simulink model "MCU_vectorControl_dsPIC33CK_LVMC_FW_teknicMotor"  (R2018a)
settings: Solver=FixedStepDiscrete  StartTime=0.0  StopTime=10.0  FixedStep=50e-6  RelTol=1e-3  EnableMultiTasking=on
undefined symbols (not defined in the file): A0, A4, AN0, AN1, B0, B2, Bias1, Bias2, C12, C13, C14, C7, control, D11, D12, D13, D14, D5, D6, D7, DiscIntNeverNeededParam, inverter, Max, MaxPer, model, ms, NumBits1, NumBits2, P20, P32, P55, P60, P61, P62, P69, P70, P71, P75, P76, P77, P78, Pin, pmsm, PosRange1, PosRange2, PWM1max, Resol, s, Slope1, Slope2, us
libraries: simulink x43, MCHP_Blockset x23
(part 4 of 4)

== system MCU_vectorControl_dsPIC33CK_LVMC_FW_teknicMotor/BOARD dsPIC33CK LVMC/Timing Analysis/Downsample Averaged2 ==
  note: DownSample & Average by changing data scaling
  In1 : Inport
  Compare To Constant : simulink/Logic and Bit Operations/Compare To Constant  relop===  const=1  OutDataTypeStr=boolean
  Counter Limited : simulink/Sources/Counter Limited  uplimit=DownSample-1  tsamp=-1
  Data Type Duplicate : DataTypeDuplicate
  Data Type Propagation : simulink/Signal Attributes/Data Type Propagation  PropDataType=fixdt(1, 16)  IfRefDouble=double  IfRefSingle=single  IsSigned=IsSigned1 or IsSigned2  NumBitsBase=NumBits1+NumBits2  NumBitsMult=1  NumBitsAdd=0  NumBitsAllowFinal=1:128  PropScaling=2^-10  ValuesUsedBestPrec=[5 -7]  SlopeBase=Slope1  SlopeMult=1  SlopeAdd=0  BiasBase=Bias1  BiasMult=1  BiasAdd=0
      settings: SourceProductName=Simulink  SourceProductBaseCode=SL
  Data Type Propagation1 : simulink/Signal Attributes/Data Type Propagation  PropDataType=fixdt(1, 16)  IfRefDouble=double  IfRefSingle=single  IsSigned=IsSigned1 or IsSigned2  NumBitsBase=NumBits1+NumBits2  NumBitsMult=1  NumBitsAdd=0  NumBitsAllowFinal=1:128  PropScaling=2^-10  ValuesUsedBestPrec=[5 -7]  SlopeBase=PosRange1  SlopeMult=1  SlopeAdd=0  BiasBase=Bias1  BiasMult=1  BiasAdd=0
      settings: SourceProductName=Simulink  SourceProductBaseCode=SL
  Discrete-Time Integrator : DiscreteIntegrator  IntegratorMethod=Accumulation: Backward Euler  gainval=1  ExternalReset=sampled level  SampleTime=-1  OutDataTypeStr=Inherit: Inherit via back propagation  ICPrevOutput=DiscIntNeverNeededParam  ICPrevScaledInput=DiscIntNeverNeededParam
  Gain : Gain  Gain=1/DownSample  OutDataTypeStr=Inherit: Inherit via back propagation
  Gain1 : Gain  Gain=1/DownSample  OutDataTypeStr=Inherit: Inherit via back propagation
  Rate Transition1 : RateTransition  Deterministic=off  OutPortSampleTime=[InputSampleTime * DownSample]
  Rate Transition3 : RateTransition  OutPortSampleTime=[InputSampleTime * DownSample]
  Terminator : Terminator
  Out1 : Outport
  wires:
  Rate Transition3/1 -> Gain1/1, Gain/1
  In1/1 -> Discrete-Time Integrator/1, Rate Transition1/1, Data Type Propagation/2, Data Type Propagation/1
  Compare To Constant/1 -> Discrete-Time Integrator/2
  Discrete-Time Integrator/1 -> Data Type Propagation/3, Rate Transition3/1
  Counter Limited/1 -> Compare To Constant/1
  Gain/1 -> Data Type Duplicate/2, Out1/1
  Rate Transition1/1 -> Data Type Propagation1/2, Data Type Propagation1/1, Data Type Duplicate/1
  Gain1/1 -> Data Type Propagation1/3, Terminator/1

== system MCU_vectorControl_dsPIC33CK_LVMC_FW_teknicMotor/Control law/Speed control/Current Control ==
  idqref : Inport
  idq : Inport  Port=2
  Data Type Duplicate : DataTypeDuplicate  NumInputPorts=3
  Data Type Propagation : simulink/Signal Attributes/Data Type Propagation  PropDataType=fixdt(1, 16)  IfRefDouble=double  IfRefSingle=single  IsSigned=IsSigned1 or IsSigned2  NumBitsBase=max([NumBits1 NumBits2])  NumBitsMult=1  NumBitsAdd=0  NumBitsAllowFinal=1:128  PropScaling=2^-(15-ceil(log2(2*inverter.iMax)))  ValuesUsedBestPrec=[5 -7]  SlopeBase=max([PosRange1 PosRange2])  SlopeMult=2  SlopeAdd=0  BiasBase=Bias1  BiasMult=1  BiasAdd=0
      settings: SourceProductName=Simulink  SourceProductBaseCode=SL
  Gain : Gain  Gain=control.kE(2)  OutDataTypeStr=Inherit: Inherit via back propagation  SaturateOnIntegerOverflow=on
  Gain1 : Gain  Gain=control.kE(1)  OutDataTypeStr=Inherit: Inherit via back propagation  SaturateOnIntegerOverflow=on
  Integrator : Subsystem
  Sum : Sum  Inputs=|--  OutDataTypeStr=Inherit: Inherit via back propagation  SaturateOnIntegerOverflow=on
  Sum3 : Sum  Inputs=|+-  OutDataTypeStr=Inherit: Inherit via back propagation  SaturateOnIntegerOverflow=on
  v : Outport
  wires:
  Sum/1 -> v/1, Data Type Duplicate/1
  Integrator/1(Out1) -> Gain/1
  idqref/1 -> Sum3/1, Data Type Propagation/1
  Sum3/1 -> Integrator/1(In1), Data Type Propagation/3
  idq/1 -> Sum3/2, Gain1/1, Data Type Propagation/2
  Gain/1 -> Sum/1, Data Type Duplicate/2
  Gain1/1 -> Sum/2, Data Type Duplicate/3

== system MCU_vectorControl_dsPIC33CK_LVMC_FW_teknicMotor/Control law/Speed control/Mechanical Control ==
  omref : Inport
  om : Inport  Port=2
  isat : Inport  Port=3
  Clamping circuit : Subsystem
  Constant : Constant  Value=0  OutMax=model.iMax  OutDataTypeStr=fixdt(1,16)
  Data Type Duplicate1 : DataTypeDuplicate
  Data Type Propagation : simulink/Signal Attributes/Data Type Propagation  PropDataType=fixdt(1, 16)  IfRefDouble=double  IfRefSingle=single  IsSigned=IsSigned1 or IsSigned2  NumBitsBase=max([NumBits1 NumBits2])  NumBitsMult=1  NumBitsAdd=0  NumBitsAllowFinal=1:128  PropScaling=2^-(15-ceil(log2(2*pmsm.omMax)))  ValuesUsedBestPrec=[5 -7]  SlopeBase=max([PosRange1 PosRange2])  SlopeMult=2  SlopeAdd=0  BiasBase=Bias1  BiasMult=1  BiasAdd=0
      settings: SourceProductName=Simulink  SourceProductBaseCode=SL
  Delay : Delay  DelayLength=1
  Gain : Gain  Gain=control.kM(2)  OutDataTypeStr=Inherit: Inherit via back propagation  SaturateOnIntegerOverflow=on
  Gain1 : Gain  Gain=control.kM(1)  OutMax=model.iMax  OutDataTypeStr=fixdt(1,16)  SaturateOnIntegerOverflow=on
  Integrator : Subsystem
  Saturation Dynamic : simulink/Discontinuities/Saturation Dynamic  OutMin=[]  OutMax=[]  OutDataTypeStr=Inherit: Same as second input  OutDataType=fixdt(1, 16)  OutScaling=2^-10  DoSatur=off
  Sum : Sum  Inputs=|--  OutMax=2*model.iMax  OutDataTypeStr=fixdt(1,16)  SaturateOnIntegerOverflow=on
  Sum1 : Sum  Inputs=|+-  OutDataTypeStr=Inherit: Inherit via back propagation
  Sum2 : Sum  Inputs=|-+  SaturateOnIntegerOverflow=on  OutDataTypeStr=Inherit: Same as first input
  iqref : Outport
  wires:
  Saturation Dynamic/1 -> Sum2/1, iqref/1
  Sum/1 -> Sum2/2, Saturation Dynamic/2
  Gain/1 -> Sum/1
  om/1 -> Sum1/2, Gain1/1, Data Type Propagation/2, Data Type Duplicate1/2
  Sum1/1 -> Integrator/1(In1), Clamping circuit/2(preIntegrator), Data Type Propagation/3
  omref/1 -> Sum1/1, Data Type Propagation/1, Data Type Duplicate1/1
  Clamping circuit/1(Clamp) -> Integrator/Enable
  Sum2/1 -> Clamping circuit/1(Saturation)
  Integrator/1(Out1) -> Gain/1
  Gain1/1 -> Sum/2
  isat/1 -> Delay/1
  Delay/1 -> Saturation Dynamic/1
  Constant/1 -> Saturation Dynamic/3

== system MCU_vectorControl_dsPIC33CK_LVMC_FW_teknicMotor/Control law/Speed control/Subsystem2 ==
  om : Inport
  iref : Inport  Port=2
  Imax : Inport  Port=3
  Subsystem6 : Subsystem
  decision1 : Subsystem
  idq : Outport  VectorParamsAs1DForOutWhenUnconnected=on
  isat : Outport  Port=2  VectorParamsAs1DForOutWhenUnconnected=on
  wires:
  om/1 -> Subsystem6/2(om)
  Imax/1 -> Subsystem6/1(Imax), decision1/1(Imax)
  iref/1 -> decision1/2(iqref)
  decision1/1(idq) -> idq/1
  Subsystem6/2(i2(w)) -> decision1/4(i2(w))
  Subsystem6/3(i4(w)) -> decision1/5(i3(w))
  Subsystem6/1(i1(w)) -> decision1/3(i1(w))
  Subsystem6/4(a(w)) -> decision1/6(a(w))
  Subsystem6/5(b(w)) -> decision1/7(b(w))
  Subsystem6/6(c(w)) -> decision1/8(c(w))
  decision1/2(isat) -> isat/1
  Subsystem6/7(delta) -> decision1/9(delta)

== system MCU_vectorControl_dsPIC33CK_LVMC_FW_teknicMotor/Control law/Voltage Saturation/Norm L3 ==
  In1 : Inport
  Data Type Propagation : simulink/Signal Attributes/Data Type Propagation  PropDataType=fixdt(1, 16)  IfRefDouble=double  IfRefSingle=single  IsSigned=IsSigned1 or IsSigned2  NumBitsBase=max([NumBits1 NumBits2])  NumBitsMult=1  NumBitsAdd=0  NumBitsAllowFinal=1:128  PropScaling=2^-10  ValuesUsedBestPrec=[5 -7]  SlopeBase=Slope1/Slope2  SlopeMult=1  SlopeAdd=0  BiasBase=max([Bias1 Bias2])  BiasMult=1  BiasAdd=0
      settings: SourceProductName=Simulink  SourceProductBaseCode=SL
  Data Type Propagation1 : simulink/Signal Attributes/Data Type Propagation  PropDataType=fixdt(1, 16)  IfRefDouble=double  IfRefSingle=single  IsSigned=IsSigned1 or IsSigned2  NumBitsBase=max([NumBits1 NumBits2])  NumBitsMult=1  NumBitsAdd=0  NumBitsAllowFinal=1:128  PropScalingMode=Specify via dialog  PropScaling=2^-(15-ceil(log2(2*model.vMax)))  ValuesUsedBestPrec=[5 -7]  SlopeBase=Slope1/Slope2  SlopeMult=1  SlopeAdd=0  BiasBase=max([Bias1 Bias2])  BiasMult=1  BiasAdd=0
      settings: SourceProductName=Simulink  SourceProductBaseCode=SL
  Dot Product : DotProduct  OutDataTypeStr=Inherit: Inherit via back propagation  SaturateOnIntegerOverflow=on  InputSameDT=on
  Sqrt : Sqrt  OutputSignalType=real  OutDataTypeStr=Inherit: Inherit via back propagation  SaturateOnIntegerOverflow=on
  y : Outport  VectorParamsAs1DForOutWhenUnconnected=on
  wires:
  Dot Product/1 -> Data Type Propagation/3, Sqrt/1
  Sqrt/1 -> y/1, Data Type Propagation1/3
  In1/1 -> Dot Product/1, Dot Product/2, Data Type Propagation/2, Data Type Propagation/1, Data Type Propagation1/1, Data Type Propagation1/2

== system MCU_vectorControl_dsPIC33CK_LVMC_FW_teknicMotor/Control law/Speed control/Current Control/Integrator ==
  In1 : Inport
  Data Type Propagation : simulink/Signal Attributes/Data Type Propagation  PropDataType=fixdt(1, 16)  IfRefDouble=single  IfRefSingle=single  IsSigned=IsSigned1 or IsSigned2  NumBitsBase=NumBits1+NumBits2  NumBitsMult=1  NumBitsAdd=0  NumBitsAllowFinal=1:128  PropScalingMode=Specify via dialog  PropScaling=2^-23  ValuesUsedBestPrec=[5 -7]  SlopeBase=min([Slope1 Slope2])  SlopeMult=1  SlopeAdd=0  BiasBase=Bias1  BiasMult=1  BiasAdd=0
      settings: SourceProductName=Simulink  SourceProductBaseCode=SL
  Discrete-Time Integrator : DiscreteIntegrator  SampleTime=-1  OutDataTypeStr=Inherit: Inherit via back propagation  SaturateOnIntegerOverflow=on  ICPrevOutput=DiscIntNeverNeededParam  ICPrevScaledInput=DiscIntNeverNeededParam
  Out1 : Outport
  wires:
  Discrete-Time Integrator/1 -> Out1/1, Data Type Propagation/3
  In1/1 -> Data Type Propagation/1, Data Type Propagation/2, Discrete-Time Integrator/1

== system MCU_vectorControl_dsPIC33CK_LVMC_FW_teknicMotor/Control law/Speed control/Mechanical Control/Clamping circuit ==
  note: The clamping enable or disable the integral action.
  Saturation : Inport  DisableCoverage=on
  preIntegrator : Inport  DisableCoverage=on  Port=2
  Compare To Zero1 : simulink/Logic and Bit Operations/Compare To Zero  relop=<=  OutDataTypeStr=boolean
  Delay : Delay  DelayLength=1  InitialCondition=0
  Multiply : Product  SaturateOnIntegerOverflow=on  OutDataTypeStr=Inherit: Same as first input
  Clamp : Outport  DisableCoverage=on
  wires:
  Delay/1 -> Multiply/1
  Saturation/1 -> Delay/1
  Multiply/1 -> Compare To Zero1/1
  preIntegrator/1 -> Multiply/2
  Compare To Zero1/1 -> Clamp/1

== system MCU_vectorControl_dsPIC33CK_LVMC_FW_teknicMotor/Control law/Speed control/Mechanical Control/Integrator ==
  In1 : Inport
  Enable : EnablePort
  Discrete-Time Integrator : DiscreteIntegrator  SampleTime=-1  OutDataTypeStr=fixdt(1,32,20)  SaturateOnIntegerOverflow=on  ICPrevOutput=DiscIntNeverNeededParam  ICPrevScaledInput=DiscIntNeverNeededParam
  Out1 : Outport
  wires:
  In1/1 -> Discrete-Time Integrator/1
  Discrete-Time Integrator/1 -> Out1/1

== system MCU_vectorControl_dsPIC33CK_LVMC_FW_teknicMotor/Control law/Speed control/Subsystem2/Subsystem6 ==
  Imax : Inport
  om : Inport  Port=2
  Compare To Constant : simulink/Logic and Bit Operations/Compare To Constant  relop=>  const=model.omBase  OutDataTypeStr=boolean
  Constant : Constant  Value=0  OutMax=model.iMax  OutDataTypeStr=fixdt(1,16)
  Contraints (9) fix : Subsystem
  Subsystem3 : Subsystem
  Subsystem4 : Subsystem
  Subsystem5 : Subsystem
  Switch : Switch  Criteria=u2 > Threshold
  i1(w) : Outport  VectorParamsAs1DForOutWhenUnconnected=on
  i2(w) : Outport  Port=2  VectorParamsAs1DForOutWhenUnconnected=on
  i4(w) : Outport  Port=3  VectorParamsAs1DForOutWhenUnconnected=on
  a(w) : Outport  Port=4  VectorParamsAs1DForOutWhenUnconnected=on
  b(w) : Outport  Port=5  VectorParamsAs1DForOutWhenUnconnected=on
  c(w) : Outport  Port=6  VectorParamsAs1DForOutWhenUnconnected=on
  delta : Outport  Port=7  VectorParamsAs1DForOutWhenUnconnected=on
  wires:
  om/1 -> Contraints (9) fix/1(om), Compare To Constant/1
  Imax/1 -> Subsystem4/4(Imax)
  Contraints (9) fix/3(c(w)) -> Subsystem5/2(c(w)), Subsystem4/3(c(w)), Subsystem3/3(c(w)), c(w)/1
  Compare To Constant/1 -> Subsystem4/Enable, Switch/2
  Subsystem4/1(i2(w)) -> Switch/1
  Contraints (9) fix/2(b(w)) -> Subsystem5/1(b(w)), Subsystem4/2(b(w)), Subsystem3/2(b(w)), b(w)/1
  Contraints (9) fix/1(a(w)) -> Subsystem3/1(a(w)), Subsystem4/1(a(w)), a(w)/1
  Subsystem3/1(i1(w)) -> i1(w)/1
  Switch/1 -> i2(w)/1
  Subsystem5/1(i4(w)) -> i4(w)/1
  Constant/1 -> Switch/3
  Subsystem4/2(delta) -> delta/1

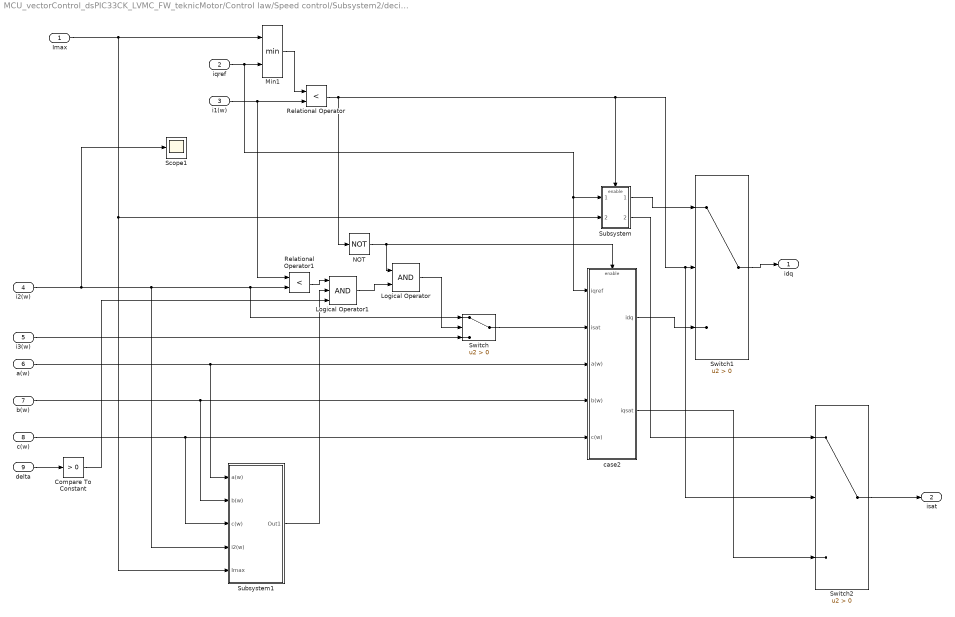
== system MCU_vectorControl_dsPIC33CK_LVMC_FW_teknicMotor/Control law/Speed control/Subsystem2/decision1 ==
  Imax : Inport
  iqref : Inport  Port=2
  i1(w) : Inport  Port=3
  i2(w) : Inport  Port=4
  i3(w) : Inport  Port=5
  a(w) : Inport  Port=6
  b(w) : Inport  Port=7
  c(w) : Inport  Port=8
  delta : Inport  Port=9
  Compare To Constant : simulink/Logic and Bit Operations/Compare To Constant  relop=>  const=0  OutDataTypeStr=boolean
  Logical Operator : Logic  AllPortsSameDT=off  OutDataTypeStr=boolean
  Logical Operator1 : Logic  Inputs=3  AllPortsSameDT=off  OutDataTypeStr=boolean
  Min1 : MinMax  Inputs=2
  NOT : Logic  Operator=NOT  IconShape=distinctive  AllPortsSameDT=off  OutDataTypeStr=boolean
  Relational Operator : RelationalOperator  Operator=<  OutDataTypeStr=boolean  RndMeth=Simplest
  Relational Operator1 : RelationalOperator  Operator=<  OutDataTypeStr=boolean  RndMeth=Simplest
  Scope1 : Scope
  Subsystem : Subsystem
  Subsystem1 : Subsystem
  Switch : Switch  Criteria=u2 > Threshold
  Switch1 : Switch  Criteria=u2 > Threshold
  Switch2 : Switch  Criteria=u2 > Threshold
  case2 : Subsystem
  idq : Outport  VectorParamsAs1DForOutWhenUnconnected=on
  isat : Outport  Port=2  VectorParamsAs1DForOutWhenUnconnected=on
  wires:
  c(w)/1 -> Subsystem1/3(c(w)), case2/5(c(w))
  b(w)/1 -> Subsystem1/2(b(w)), case2/4(b(w))
  a(w)/1 -> Subsystem1/1(a(w)), case2/3(a(w))
  i3(w)/1 -> Switch/3
  iqref/1 -> Subsystem/1(iref), case2/1(iqref), Min1/2
  Logical Operator/1 -> Switch/2
  NOT/1 -> case2/Enable, Logical Operator/1
  Subsystem/1(idq) -> Switch1/1
  i1(w)/1 -> Relational Operator/2, Relational Operator1/1
  Switch1/1 -> idq/1
  case2/1(idq) -> Switch1/3
  Relational Operator/1 -> Switch2/2, Switch1/2, Subsystem/Enable, NOT/1
  Min1/1 -> Relational Operator/1
  Subsystem1/1(Out1) -> Logical Operator1/2
  Imax/1 -> Subsystem/2(iMax), Subsystem1/5(Imax), Min1/1
  Relational Operator1/1 -> Logical Operator1/1
  Logical Operator1/1 -> Logical Operator/2
  i2(w)/1 -> Scope1/1, Subsystem1/4(i2(w)), Relational Operator1/2, Switch/1
  Switch/1 -> case2/2(isat)
  delta/1 -> Compare To Constant/1
  Compare To Constant/1 -> Logical Operator1/3
  Subsystem/2(iqsat) -> Switch2/1
  case2/2(iqsat) -> Switch2/3
  Switch2/1 -> isat/1

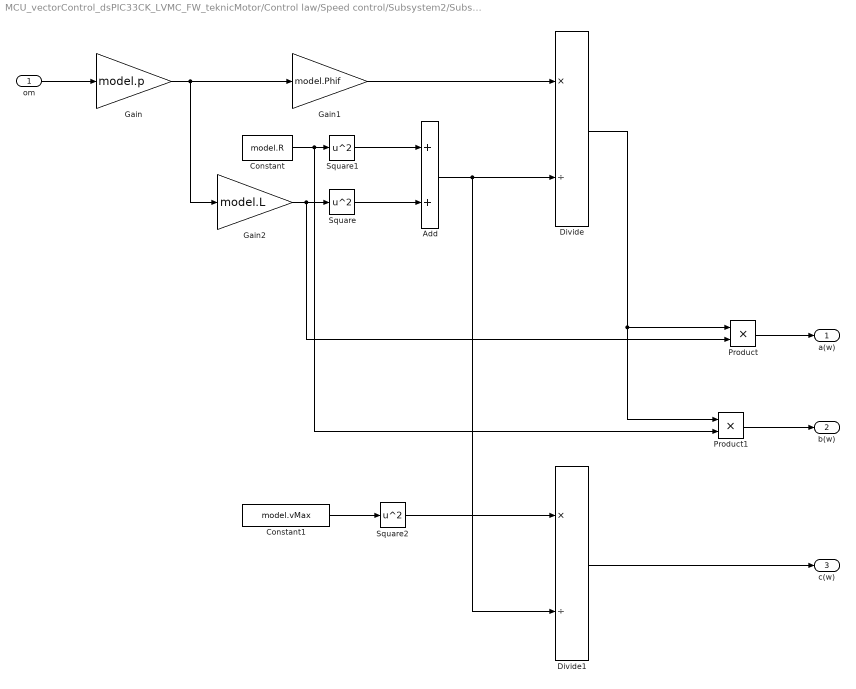
== system MCU_vectorControl_dsPIC33CK_LVMC_FW_teknicMotor/Control law/Speed control/Subsystem2/Subsystem6/Contraints (9) fix ==
  om : Inport
  Add : Sum  OutMax=(model.R.^2+(model.p*model.omMax*model.L).^2)  OutDataTypeStr=fixdt(0,16)  SaturateOnIntegerOverflow=on
  Constant : Constant  Value=model.R  OutMax=model.R  OutDataTypeStr=fixdt(0,16)
  Constant1 : Constant  Value=model.vMax  OutMax=model.vMax  OutDataTypeStr=fixdt(0,16)
  Divide : Product  Inputs=*/  OutMax=max((model.p*(0:0.1:model.omMax)*model.Phif./(model.R.^2+(model.p*(0:0.1:model.omMax)*model.L).^2)))  OutDataTypeStr=fixdt(0,16)
  Divide1 : Product  Inputs=*/  OutMax=max((model.vMax*model.vMax./(model.R.^2+(model.p*(0:0.1:model.omMax)*model.L).^2)))  OutDataTypeStr=fixdt(0,16)  SaturateOnIntegerOverflow=on
  Gain : Gain  Gain=model.p  OutMax=model.p*model.omMax  OutDataTypeStr=fixdt(0,16)
  Gain1 : Gain  Gain=model.Phif  OutMax=model.p*model.Phif*model.omMax  OutDataTypeStr=fixdt(0,16)  SaturateOnIntegerOverflow=on
  Gain2 : Gain  Gain=model.L  OutMax=model.L*model.p*model.omMax  OutDataTypeStr=fixdt(0,16)  SaturateOnIntegerOverflow=on
  Product : Product  OutMax=model.L*model.p*model.omMax*max((model.p*(0:0.1:model.omMax)*model.Phif./(model.R.^2+(model.p*(0:0.1:model.omMax)*model.L).^2)))  OutDataTypeStr=fixdt(0,16)  SaturateOnIntegerOverflow=on
  Product1 : Product  OutMax=model.R*max((model.p*(0:0.1:model.omMax)*model.Phif./(model.R.^2+(model.p*(0:0.1:model.omMax)*model.L).^2)))  OutDataTypeStr=fixdt(0,16)  SaturateOnIntegerOverflow=on
  Square : Math  Operator=square  OutMax=(model.L*model.p*model.omMax)^2  OutDataTypeStr=fixdt(0,16)  SaturateOnIntegerOverflow=on
  Square1 : Math  Operator=square  OutMax=model.R*model.R  OutDataTypeStr=fixdt(0,16)  SaturateOnIntegerOverflow=on
  Square2 : Math  Operator=square  OutMax=model.vMax*model.vMax  OutDataTypeStr=fixdt(0,16)  SaturateOnIntegerOverflow=on
  a(w) : Outport  VectorParamsAs1DForOutWhenUnconnected=on
  b(w) : Outport  Port=2  VectorParamsAs1DForOutWhenUnconnected=on
  c(w) : Outport  Port=3  VectorParamsAs1DForOutWhenUnconnected=on
  wires:
  Product1/1 -> b(w)/1
  Square1/1 -> Add/1
  Gain1/1 -> Divide/1
  Constant1/1 -> Square2/1
  Product/1 -> a(w)/1
  Square/1 -> Add/2
  om/1 -> Gain/1
  Constant/1 -> Product1/2, Square1/1
  Divide/1 -> Product1/1, Product/1
  Add/1 -> Divide1/2, Divide/2
  Gain2/1 -> Product/2, Square/1
  Gain/1 -> Gain2/1, Gain1/1
  Divide1/1 -> c(w)/1
  Square2/1 -> Divide1/1

== system MCU_vectorControl_dsPIC33CK_LVMC_FW_teknicMotor/Control law/Speed control/Subsystem2/Subsystem6/Subsystem3 ==
  a(w) : Inport
  b(w) : Inport  Port=2
  c(w) : Inport  Port=3
  Add : Sum  Inputs=+-  SaturateOnIntegerOverflow=on  OutDataTypeStr=Inherit: Same as first input
  Add1 : Sum  Inputs=+-  OutMax=model.iMax  OutDataTypeStr=fixdt(1,16)  SaturateOnIntegerOverflow=on
  Constant1 : Constant  Value=0  OutDataTypeStr=int16
  Sqrt : Sqrt  SaturateOnIntegerOverflow=on
  Square : Math  Operator=square  OutMax=(model.L*model.p*model.omMax*max((model.p*(0:0.1:model.omMax)*model.Phif./(model.R.^2+(model.p*(0:0.1:model.omMax)*model.L).^2)))).^2  OutDataTypeStr=fixdt(0,16)  SaturateOnIntegerOverflow=on
  Switch2 : Switch  Criteria=u2 > Threshold
  Switch3 : Switch  Criteria=u2 > Threshold
  i1(w) : Outport  VectorParamsAs1DForOutWhenUnconnected=on
  wires:
  Add1/1 -> Switch3/1
  Square/1 -> Add/2
  a(w)/1 -> Square/1
  c(w)/1 -> Add/1
  b(w)/1 -> Add1/2
  Sqrt/1 -> Add1/1
  Add/1 -> Switch2/1, Switch3/2, Switch2/2
  Constant1/1 -> Switch3/3, Switch2/3
  Switch2/1 -> Sqrt/1
  Switch3/1 -> i1(w)/1

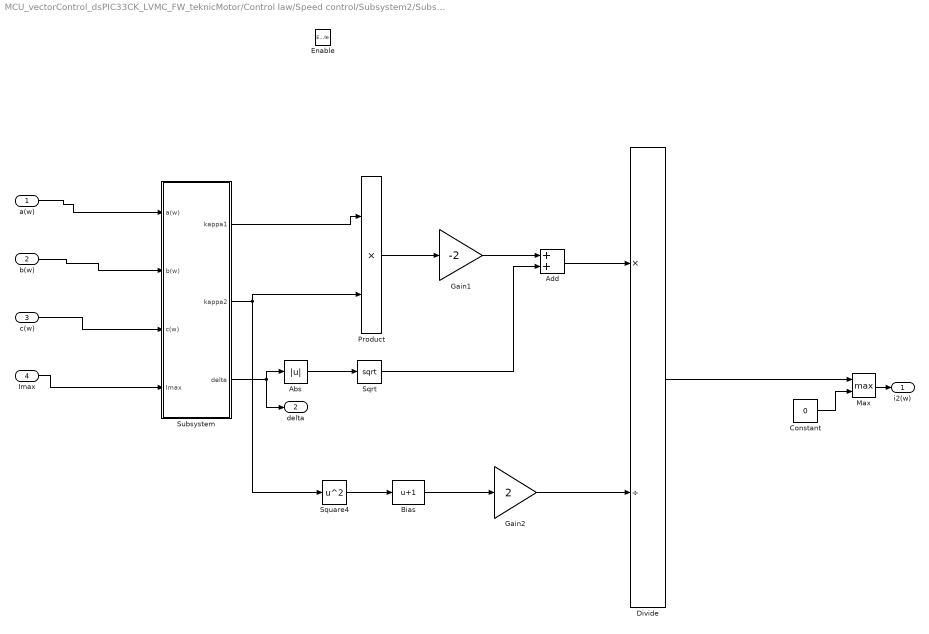
== system MCU_vectorControl_dsPIC33CK_LVMC_FW_teknicMotor/Control law/Speed control/Subsystem2/Subsystem6/Subsystem4 ==
  a(w) : Inport
  b(w) : Inport  Port=2
  c(w) : Inport  Port=3
  Imax : Inport  Port=4
  Enable : EnablePort
  Abs : Abs
  Add : Sum  OutMax=[2*model.iMax^2]  OutDataTypeStr=fixdt(1,16)
  Bias : Bias  Bias=1
  Constant : Constant  Value=0  OutMax=[model.iMax]  OutDataTypeStr=fixdt(1,16)
  Divide : Product  Inputs=*/  OutMax=[model.iMax]  OutDataTypeStr=fixdt(1,16)
  Gain1 : Gain  Gain=-2  OutMax=[model.iMax^2]  OutDataTypeStr=fixdt(1,16)
  Gain2 : Gain  Gain=2  OutMax=[2*model.iMax^2]  OutDataTypeStr=fixdt(1,16)
  Max : MinMax  Function=max  Inputs=2
  Product : Product  OutMax=model.iMax*model.iMax  OutDataTypeStr=fixdt(1,16)
  Sqrt : Sqrt  OutMax=[4*model.iMax^2]  OutDataTypeStr=fixdt(1,16)  SaturateOnIntegerOverflow=on
  Square4 : Math  Operator=square  OutMax=[model.iMax^2]  OutDataTypeStr=fixdt(1,16)  SaturateOnIntegerOverflow=on
  Subsystem : Subsystem
  i2(w) : Outport  VectorParamsAs1DForOutWhenUnconnected=on
  delta : Outport  Port=2  VectorParamsAs1DForOutWhenUnconnected=on
  wires:
  Subsystem/3(delta) -> Abs/1, delta/1
  Subsystem/2(kappa2) -> Product/2, Square4/1
  Max/1 -> i2(w)/1
  Bias/1 -> Gain2/1
  Constant/1 -> Max/2
  Square4/1 -> Bias/1
  Gain1/1 -> Add/1
  Gain2/1 -> Divide/2
  Sqrt/1 -> Add/2
  Product/1 -> Gain1/1
  Add/1 -> Divide/1
  Divide/1 -> Max/1
  Imax/1 -> Subsystem/4(Imax)
  c(w)/1 -> Subsystem/3(c(w))
  b(w)/1 -> Subsystem/2(b(w))
  a(w)/1 -> Subsystem/1(a(w))
  Abs/1 -> Sqrt/1
  Subsystem/1(kappa1) -> Product/1

== system MCU_vectorControl_dsPIC33CK_LVMC_FW_teknicMotor/Control law/Speed control/Subsystem2/Subsystem6/Subsystem5 ==
  b(w) : Inport
  c(w) : Inport  Port=2
  Add : Sum  Inputs=+-  OutMax=2*model.iMax  OutDataTypeStr=fixdt(0,16)  SaturateOnIntegerOverflow=on
  Sqrt : Sqrt  OutMax=2*model.iMax  OutDataTypeStr=fixdt(0,16)  SaturateOnIntegerOverflow=on
  i4(w) : Outport  VectorParamsAs1DForOutWhenUnconnected=on
  wires:
  b(w)/1 -> Add/2
  Sqrt/1 -> Add/1
  c(w)/1 -> Sqrt/1
  Add/1 -> i4(w)/1

== system MCU_vectorControl_dsPIC33CK_LVMC_FW_teknicMotor/Control law/Speed control/Subsystem2/decision1/Subsystem ==
  iref : Inport
  iMax : Inport  Port=2
  Enable : EnablePort
  Constant : Constant  Value=0  OutMax=model.iMax  OutDataTypeStr=fixdt(1,16)
  Min : MinMax  Inputs=2
  Mux : Mux  Inputs=2
  idq : Outport  VectorParamsAs1DForOutWhenUnconnected=on
  iqsat : Outport  Port=2  VectorParamsAs1DForOutWhenUnconnected=on
  wires:
  Constant/1 -> Mux/1
  Min/1 -> Mux/2
  iref/1 -> Min/1
  Mux/1 -> idq/1
  iMax/1 -> iqsat/1, Min/2

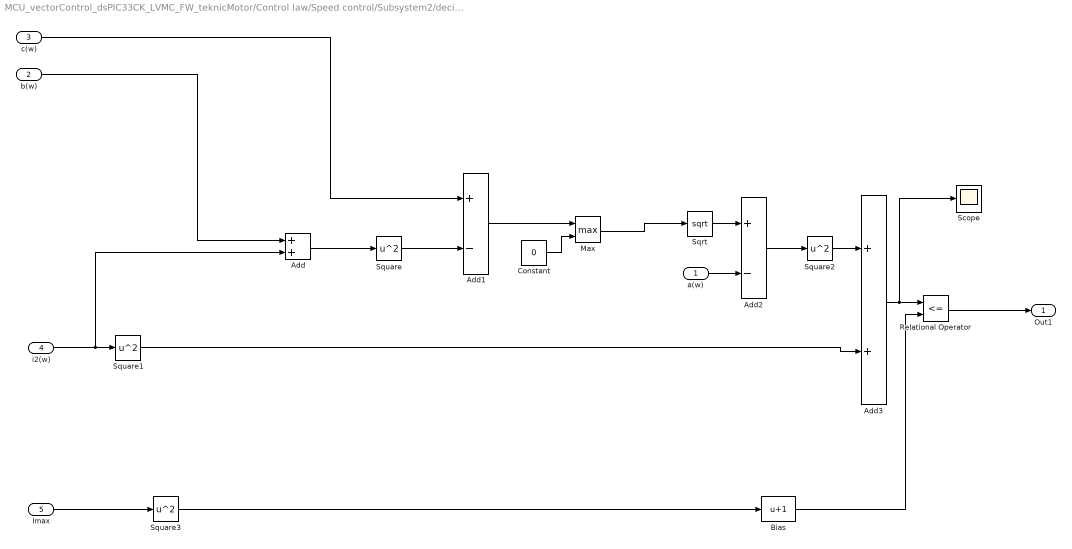
== system MCU_vectorControl_dsPIC33CK_LVMC_FW_teknicMotor/Control law/Speed control/Subsystem2/decision1/Subsystem1 ==
  a(w) : Inport
  b(w) : Inport  Port=2
  c(w) : Inport  Port=3
  i2(w) : Inport  Port=4
  Imax : Inport  Port=5
  Add : Sum  OutMax=2*model.iMax  OutDataTypeStr=fixdt(1,16)  SaturateOnIntegerOverflow=on
  Add1 : Sum  Inputs=+-  SaturateOnIntegerOverflow=on
  Add2 : Sum  Inputs=+-  OutMax=model.iMax  OutDataTypeStr=fixdt(1,16)  SaturateOnIntegerOverflow=on
  Add3 : Sum  OutMax=4*model.iMax*model.iMax  OutDataTypeStr=fixdt(1,16)  SaturateOnIntegerOverflow=on
  Bias : Bias  Bias=1  SaturateOnIntegerOverflow=on
  Constant : Constant  Value=0  OutDataTypeStr=int16
  Max : MinMax  Function=max  Inputs=2  SaturateOnIntegerOverflow=on
  Relational Operator : RelationalOperator  Operator=<=  OutDataTypeStr=boolean  RndMeth=Simplest
  Scope : Scope
  Sqrt : Sqrt  OutMax=model.iMax  OutDataTypeStr=fixdt(1,16)  SaturateOnIntegerOverflow=on
  Square : Math  Operator=square  OutMax=2*model.iMax*model.iMax  OutDataTypeStr=fixdt(1,16)  SaturateOnIntegerOverflow=on
  Square1 : Math  Operator=square  OutMax=model.iMax*model.iMax  OutDataTypeStr=fixdt(1,16)  SaturateOnIntegerOverflow=on
  Square2 : Math  Operator=square  OutMax=model.iMax*model.iMax  OutDataTypeStr=fixdt(1,16)  SaturateOnIntegerOverflow=on
  Square3 : Math  Operator=square  OutMax=model.iMax*model.iMax  OutDataTypeStr=fixdt(1,16)  SaturateOnIntegerOverflow=on
  Out1 : Outport  VectorParamsAs1DForOutWhenUnconnected=on
  wires:
  Add/1 -> Square/1
  b(w)/1 -> Add/1
  Sqrt/1 -> Add2/1
  c(w)/1 -> Add1/1
  i2(w)/1 -> Add/2, Square1/1
  Square/1 -> Add1/2
  Add2/1 -> Square2/1
  Square1/1 -> Add3/2
  a(w)/1 -> Add2/2
  Square2/1 -> Add3/1
  Add3/1 -> Scope/1, Relational Operator/1
  Imax/1 -> Square3/1
  Square3/1 -> Bias/1
  Bias/1 -> Relational Operator/2
  Relational Operator/1 -> Out1/1
  Add1/1 -> Max/1
  Constant/1 -> Max/2
  Max/1 -> Sqrt/1

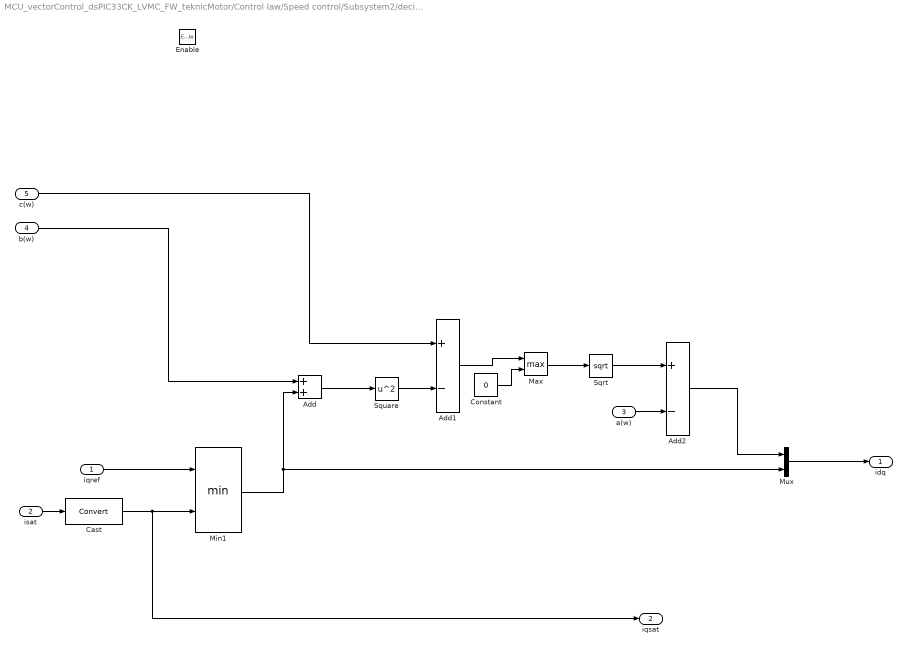
== system MCU_vectorControl_dsPIC33CK_LVMC_FW_teknicMotor/Control law/Speed control/Subsystem2/decision1/case2 ==
  iqref : Inport
  isat : Inport  Port=2
  a(w) : Inport  Port=3
  b(w) : Inport  Port=4
  c(w) : Inport  Port=5
  Enable : EnablePort
  Add : Sum  OutMax=2*model.iMax  OutDataTypeStr=fixdt(0,16)  SaturateOnIntegerOverflow=on
  Add1 : Sum  Inputs=+-  AccumDataTypeStr=fixdt(1,32,20)  OutMax=model.iMax*model.iMax  OutDataTypeStr=fixdt(1,16)  SaturateOnIntegerOverflow=on
  Add2 : Sum  Inputs=+-  OutMax=model.iMax  OutDataTypeStr=fixdt(1,16)  SaturateOnIntegerOverflow=on
  Cast : DataTypeConversion
  Constant : Constant  Value=0  OutDataTypeStr=int16
  Max : MinMax  Function=max  Inputs=2  SaturateOnIntegerOverflow=on
  Min1 : MinMax  Inputs=2  SaturateOnIntegerOverflow=on
  Mux : Mux  Inputs=2
  Sqrt : Sqrt  OutMax=model.iMax  OutDataTypeStr=fixdt(1,16)  SaturateOnIntegerOverflow=on
  Square : Math  Operator=square  OutMax=3*model.iMax*model.iMax  OutDataTypeStr=fixdt(0,16)  SaturateOnIntegerOverflow=on
  idq : Outport  VectorParamsAs1DForOutWhenUnconnected=on
  iqsat : Outport  Port=2  VectorParamsAs1DForOutWhenUnconnected=on
  wires:
  Add2/1 -> Mux/1
  Mux/1 -> idq/1
  a(w)/1 -> Add2/2
  Sqrt/1 -> Add2/1
  Add1/1 -> Max/1
  c(w)/1 -> Add1/1
  Square/1 -> Add1/2
  Add/1 -> Square/1
  b(w)/1 -> Add/1
  iqref/1 -> Min1/1
  isat/1 -> Cast/1
  Min1/1 -> Add/2, Mux/2
  Max/1 -> Sqrt/1
  Constant/1 -> Max/2
  Cast/1 -> iqsat/1, Min1/2

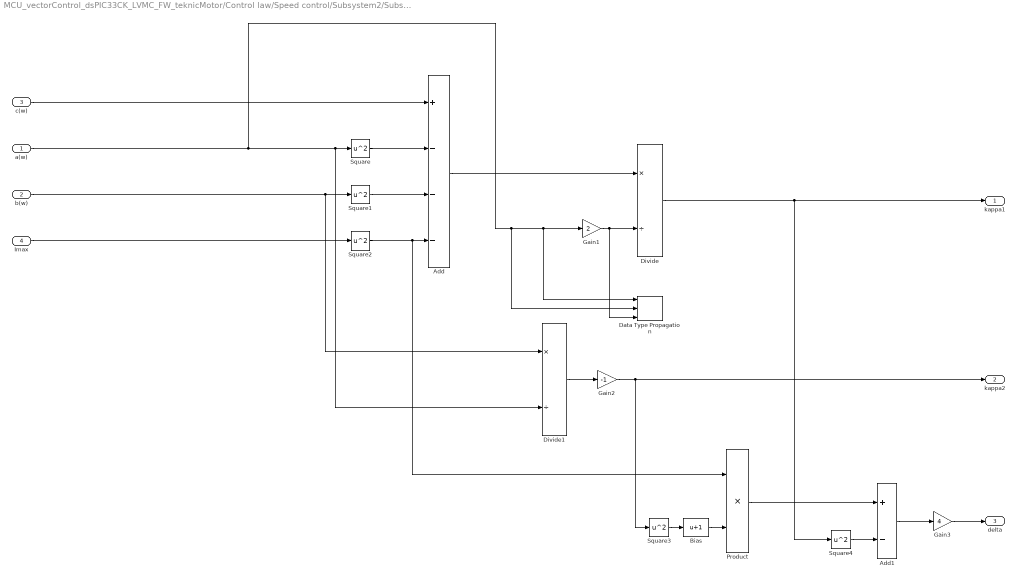
== system MCU_vectorControl_dsPIC33CK_LVMC_FW_teknicMotor/Control law/Speed control/Subsystem2/Subsystem6/Subsystem4/Subsystem ==
  a(w) : Inport
  b(w) : Inport  Port=2
  c(w) : Inport  Port=3
  Imax : Inport  Port=4
  Add : Sum  Inputs=+---  AccumDataTypeStr=fixdt(1,32,22)  OutMax=[3*model.iMax*model.iMax]  OutDataTypeStr=fixdt(1,32)  SaturateOnIntegerOverflow=on
  Add1 : Sum  Inputs=+-
  Bias : Bias  Bias=1
  Data Type Propagation : simulink/Signal Attributes/Data Type Propagation  PropDataType=fixdt(1, 16)  IfRefDouble=double  IfRefSingle=single  IsSigned=IsSigned1 or IsSigned2  NumBitsBase=max([NumBits1 NumBits2])  NumBitsMult=1  NumBitsAdd=0  NumBitsAllowFinal=1:128  PropScaling=2^-10  ValuesUsedBestPrec=[5 -7]  SlopeBase=max([Slope1 Slope2])  SlopeMult=2  SlopeAdd=0  BiasBase=Bias1  BiasMult=1  BiasAdd=0
      settings: SourceProductName=Simulink  SourceProductBaseCode=SL
  Divide : Product  Inputs=*/  OutMax=[2*model.iMax]  OutDataTypeStr=fixdt(1,16)
  Divide1 : Product  Inputs=*/  OutMax=model.iMax  OutDataTypeStr=fixdt(1,16)
  Gain1 : Gain  Gain=2  OutDataTypeStr=Inherit: Inherit via back propagation
  Gain2 : Gain  Gain=-1  OutDataTypeStr=Inherit: Same as input
  Gain3 : Gain  Gain=4  OutMax=[4*model.iMax^3]  OutDataTypeStr=fixdt(1,16)
  Product : Product  OutMax=[model.iMax^3]  OutDataTypeStr=fixdt(1,16)
  Square : Math  Operator=square  OutMax=(model.L*model.p*model.omMax*max((model.p*(0:0.1:model.omMax)*model.Phif./(model.R.^2+(model.p*(0:0.1:model.omMax)*model.L).^2)))).^2  OutDataTypeStr=fixdt(0,16)  SaturateOnIntegerOverflow=on
  Square1 : Math  Operator=square  OutMax=(model.R*max((model.p*(0:0.1:model.omMax)*model.Phif./(model.R.^2+(model.p*(0:0.1:model.omMax)*model.L).^2))))^2  OutDataTypeStr=fixdt(0,16)  SaturateOnIntegerOverflow=on
  Square2 : Math  Operator=square  OutMax=model.iMax^2  OutDataTypeStr=fixdt(0,16)  SaturateOnIntegerOverflow=on
  Square3 : Math  Operator=square  SaturateOnIntegerOverflow=on
  Square4 : Math  Operator=square  OutMax=[model.iMax^3]  OutDataTypeStr=fixdt(1,16)  SaturateOnIntegerOverflow=on
  kappa1 : Outport  VectorParamsAs1DForOutWhenUnconnected=on
  kappa2 : Outport  Port=2  VectorParamsAs1DForOutWhenUnconnected=on
  delta : Outport  Port=3  VectorParamsAs1DForOutWhenUnconnected=on
  wires:
  b(w)/1 -> Square1/1, Divide1/1
  Imax/1 -> Square2/1
  c(w)/1 -> Add/1
  Square1/1 -> Add/3
  Square/1 -> Add/2
  Gain2/1 -> Square3/1, kappa2/1
  Square2/1 -> Add/4, Product/1
  Divide/1 -> Square4/1, kappa1/1
  Product/1 -> Add1/1
  Square3/1 -> Bias/1
  Divide1/1 -> Gain2/1
  Gain3/1 -> delta/1
  Add/1 -> Divide/1
  Add1/1 -> Gain3/1
  Square4/1 -> Add1/2
  Bias/1 -> Product/2
  Gain1/1 -> Data Type Propagation/3, Divide/2
  a(w)/1 -> Divide1/2, Square/1, Data Type Propagation/2, Data Type Propagation/1, Gain1/1
